simulink model "llc_converter"  (R2025b)
settings: Solver=VariableStepAuto  StartTime=0.0  StopTime=0.001  RelTol=1e-3
libraries: spsSeriesRLCBranchLib x5, spsDiodeLib x4, spsMosfetLib x4, spsVoltageMeasurementLib x3, spsCurrentMeasurementLib x2, spsDCVoltageSourceLib x1, spsLinearTransformerLib x1, sps_lib x1
settings Model: Creator=som  LastModifiedBy=som

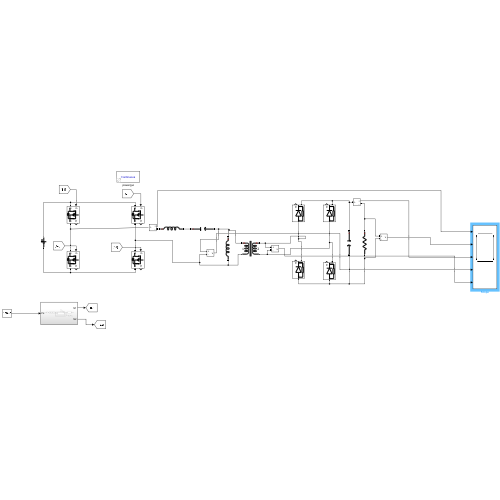
[thumbnail: Simulink's stored preview of the top-level diagram]
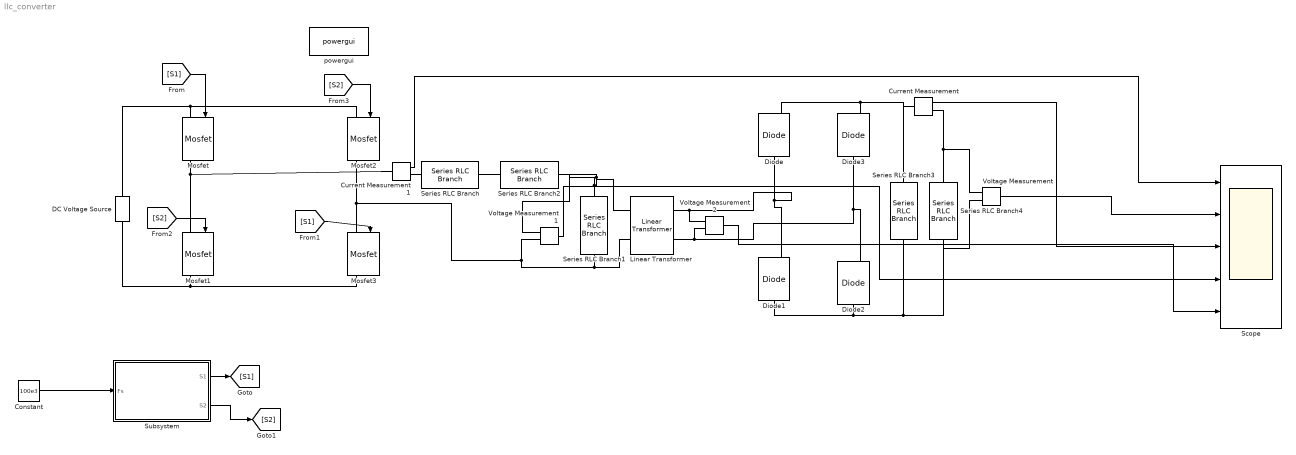
== system llc_converter ==
  Constant : Constant  Value=100e3
  Current Measurement : spsCurrentMeasurementLib/Current Measurement  PhasorSimulation=off  OutputType=Complex  PSBequivalent=0
  Current Measurement1 : spsCurrentMeasurementLib/Current Measurement  PhasorSimulation=off  OutputType=Complex  PSBequivalent=0
  DC Voltage Source : spsDCVoltageSourceLib/DC Voltage Source  Amplitude=300  Measurements=Voltage
  Diode{,1..3} (4 alike) : spsDiodeLib/Diode  Ron=0.001  Lon=0  Vf=0.8  IC=0  UseSnubber=0  Rs=500  Cs=250e-9  Measurements=on
  Linear Transformer : spsLinearTransformerLib/Linear Transformer  UNITS=SI  NominalPower=[700 100e3]  winding1=[3 0 0]  winding2=[1 0 0]  ThreeWindings=off  winding3=[3.15e+05 0.7938 0.084225]  RmLm=[100 0]  Measurements=None  DataType=on
  Mosfet{,1..3} (4 alike) : spsMosfetLib/Mosfet  Ron=0.1  Lon=0  Rd=0.01  Vfd=0  IC=0  Rs=1e5  Cs=inf  Measurements=on
  Scope : Scope  NumInputPorts=5
      settings: ActiveDisplayYMinimum=-8.6789159501921649  ActiveDisplayYMaximum=-6.6789159501921649
  Series RLC Branch : spsSeriesRLCBranchLib/Series RLC Branch  LConnTagsString=__new0  RConnTagsString=__new0  BranchType=L  Resistance=1  Inductance=22.6e-6  SetiL0=off  InitialCurrent=0  Capacitance=1e-6  Setx0=off  InitialVoltage=0  Measurements=None
  Series RLC Branch1 : spsSeriesRLCBranchLib/Series RLC Branch  LConnTagsString=__new0  RConnTagsString=__new0  BranchType=L  Resistance=1  Inductance=3.5*22.6e-6  SetiL0=off  InitialCurrent=0  Capacitance=1e-6  Setx0=off  InitialVoltage=0  Measurements=None
  Series RLC Branch2 : spsSeriesRLCBranchLib/Series RLC Branch  LConnTagsString=__new0  RConnTagsString=__new0  BranchType=C  Resistance=1  Inductance=1e-3  SetiL0=off  InitialCurrent=0  Capacitance=112e-9  Setx0=off  InitialVoltage=0  Measurements=None
  Series RLC Branch3 : spsSeriesRLCBranchLib/Series RLC Branch  LConnTagsString=__new0  RConnTagsString=__new0  BranchType=C  Resistance=1  Inductance=1e-3  SetiL0=off  InitialCurrent=0  Capacitance=100e-6  Setx0=off  InitialVoltage=0  Measurements=None
  Series RLC Branch4 : spsSeriesRLCBranchLib/Series RLC Branch  LConnTagsString=__new0  RConnTagsString=__new0  BranchType=R  Resistance=5000  Inductance=1e-3  SetiL0=off  InitialCurrent=0  Capacitance=1e-6  Setx0=off  InitialVoltage=0  Measurements=None
  Subsystem : Subsystem
  Voltage Measurement : spsVoltageMeasurementLib/Voltage Measurement  PhasorSimulation=off  OutputType=Complex  PSBequivalent=0
  Voltage Measurement1 : spsVoltageMeasurementLib/Voltage Measurement  PhasorSimulation=off  OutputType=Complex  PSBequivalent=0
  Voltage Measurement2 : spsVoltageMeasurementLib/Voltage Measurement  PhasorSimulation=off  OutputType=Complex  PSBequivalent=0
  powergui : sps_lib/powergui  Priority=1  SimulationMode=Continuous  SampleTime=50e-6  frequency=60  Iterations=50  frequencyindice=0  Pbase=100e6  ErrMax=1e-4  UnitsV=kV  UnitsW=MW  buscounter=0  FunctionMessages=off  echomessages=off  EnableUseOfTLC=off  CurrentSourceSwitches=off  DisableSnubberDevices=off  DisableRonSwitches=off  DisableVfSwitches=off  DisplayEquations=off  AutomaticDiscreteSolvers=off  SolverType=Tustin/Backward Euler (TBE)  Interpol=off  ExternalGateDelay=off  methode=off  Ts=100  x0status=blocks  SPID=on  SwTol=0  HookPort=off  NonlinearTolerance=1e-4  nMaxIteration=100  ContinueOnMaxIteration=off  RestoreLinks=warning  ResistiveCurrentMeasurement=off  Frange=[0:2:500]  Ylog=off  Xlog=on  ShowGrid=off  save=off  variable=ZData  structure=0  ZoomFFT=off  StartTime=0.0  cycles=1  DisplayStyle=1  fundamental=60  FreqAxis=off  MaxFrequency=1000  frequencyindicesteady=1  RmsSteady=1  display=off
  wires:
  Voltage Measurement/1 -> Scope/2
  Constant/1 -> Subsystem/1(Fs)
  Subsystem/2(S2) -> [S2]
  Subsystem/1(S1) -> [S1]
  [S1] -> Mosfet/1
  [S1] -> Mosfet3/1
  [S2] -> Mosfet1/1
  [S2] -> Mosfet2/1
  Voltage Measurement1/1 -> Scope/4
  Current Measurement1/1 -> Scope/1
  Current Measurement/1 -> Scope/3
  Voltage Measurement2/1 -> Scope/5
  connections:
  DC Voltage Source/RConn1 -- Mosfet2/LConn1 -- Mosfet/LConn1
  DC Voltage Source/LConn1 -- Mosfet3/RConn1 -- Mosfet1/RConn1
  Mosfet1/LConn1 -- Current Measurement1/LConn1 -- Mosfet/RConn1
  Series RLC Branch2/LConn1 -- Series RLC Branch/RConn1
  Series RLC Branch1/LConn1 -- Voltage Measurement1/LConn1 -- Series RLC Branch2/RConn1 -- Linear Transformer/LConn1
  Diode3/RConn1 -- Series RLC Branch3/LConn1 -- Current Measurement/LConn1 -- Diode/RConn1
  Diode1/LConn1 -- Voltage Measurement/LConn2 -- Series RLC Branch4/RConn1 -- Series RLC Branch3/RConn1 -- Diode2/LConn1
  Diode1/RConn1 -- Diode/LConn1 -- Voltage Measurement2/LConn1 -- Linear Transformer/RConn1
  Diode2/RConn1 -- Voltage Measurement2/LConn2 -- Linear Transformer/RConn2 -- Diode3/LConn1
  Voltage Measurement/LConn1 -- Current Measurement/RConn1 -- Series RLC Branch4/LConn1
  Series RLC Branch1/RConn1 -- Mosfet3/LConn1 -- Mosfet2/RConn1 -- Voltage Measurement1/LConn2 -- Linear Transformer/LConn2
  Series RLC Branch/LConn1 -- Current Measurement1/RConn1

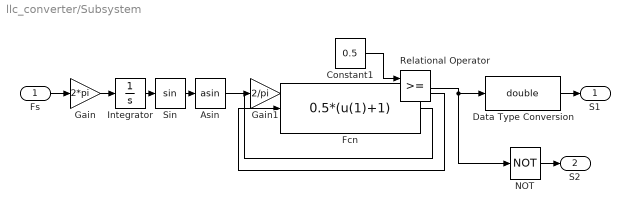
== system llc_converter/Subsystem ==
  Fs : Inport
  Asin : Trigonometry  Operator=asin
  Constant1 : Constant  Value=0.5
  Data Type Conversion : DataTypeConversion  OutDataTypeStr=double  SaturateOnIntegerOverflow=off  RndMeth=Floor
  Fcn : Fcn  Expr=0.5*(u(1)+1)
  Gain : Gain  Gain=2*pi
  Gain1 : Gain  Gain=2/pi
  Integrator : Integrator
  NOT : Logic  Operator=NOT  IconShape=distinctive  AllPortsSameDT=off  OutDataTypeStr=boolean
  Relational Operator : RelationalOperator  OutDataTypeStr=boolean  RndMeth=Simplest  InputSameDT=off
  Sin : Trigonometry
  S1 : Outport
  S2 : Outport  Port=2
  wires:
  Gain1/1 -> Fcn/1
  Asin/1 -> Gain1/1
  Gain/1 -> Integrator/1
  Integrator/1 -> Sin/1
  Fcn/1 -> Relational Operator/2
  Data Type Conversion/1 -> S1/1
  Sin/1 -> Asin/1
  Constant1/1 -> Relational Operator/1
  Relational Operator/1 -> NOT/1, Data Type Conversion/1
  Fs/1 -> Gain/1
  NOT/1 -> S2/1
